simulink model "ESPp_linear_stiff"  (R2020b)
settings: Solver=ode8  StartTime=0.0  StopTime=T  FixedStep=0.001  RelTol=1e-3
values from neighbouring files (symbols this model uses):
  D = diag([d_par d_par d_par])    [main.m]    (also in main_linear.m)
  F = 1000*[-sin(q0(1)+q0(2)+q0(3)); cos(q0(1)+q0(2)+q0(3))]    [main.m]    (also in main_linear.m)
  invB = inv(B)    [main.m]    (also in main_linear.m)
  Kd = diag([500 500 500])    [main.m]    (also in main_linear.m = diag([kd_par kd_par kd_par]))
  Kp = diag([800 800 800])    [main.m]    (also in main_linear.m = diag([kp_par kp_par kp_par]))
  link = 3    [main.m]    (also in main_linear.m)
  motor = [I_m*k_r^2, k]    [main.m]    (also in main_linear.m = [I_m*k_r^2, k, k_new])
  param = [m mm d I g0]'    [main.m]    (also in main_linear.m)
  q0 = qd    [main.m]    (also in main_linear.m)
  qd = [pi/2; 0; 0]    [main.m]    (also in main_linear.m = [pi/3; -pi/7; pi/4])
  qd0 = [0; 0; 0]    [main.m]    (also in main_linear.m)
  qd_2dot = [0; 0; 0]    [main.m]    (also in main_linear.m)
  qd_3dot = [0; 0; 0]    [main.m]    (also in main_linear.m)
  qd_4dot = [0; 0; 0]    [main.m]    (also in main_linear.m)
  qd_dot = [0; 0; 0]    [main.m]    (also in main_linear.m)
  T1 = 2    [main.m]    (also in main_linear.m)
  T2 = 3    [main.m]    (also in main_linear.m)
  theta0 = q0    [main.m]    (also in main_linear.m)
  thetad0 = [0; 0; 0]    [main.m]    (also in main_linear.m)
settings Model: Creator=lorenzo  LastModifiedBy=lorenzo

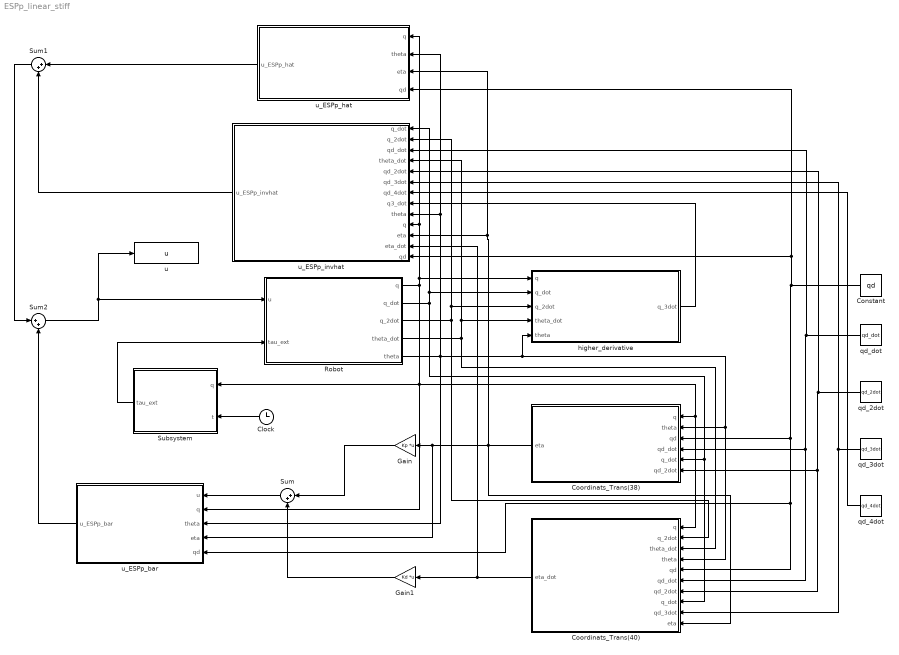
== system ESPp_linear_stiff ==
  Clock : Clock
  Constant : Constant  Value=qd  VectorParams1D=off
  Coordinats_Trans(38) : Subsystem
  Coordinats_Trans(40) : Subsystem
  Gain : Gain  Gain=Kp  Multiplication=Matrix(K*u) (u vector)
  Gain1 : Gain  Gain=Kd  Multiplication=Matrix(K*u) (u vector)
  Robot : Subsystem
  Subsystem : Subsystem
  Sum : Sum  Inputs=|++
  Sum1 : Sum  Inputs=|++
  Sum2 : Sum  Inputs=|++
  higher_derivative : Subsystem
  qd_2dot : Constant  Value=qd_2dot  VectorParams1D=off
  qd_3dot : Constant  Value=qd_3dot  VectorParams1D=off
  qd_4dot : Constant  Value=qd_4dot  VectorParams1D=off
  qd_dot : Constant  Value=qd_dot  VectorParams1D=off
  u : ToWorkspace  VariableName=u  SampleTime=-1
  u_ESPp_bar : Subsystem
  u_ESPp_hat : Subsystem
  u_ESPp_invhat : Subsystem
  wires:
  Robot/1(q) -> u_ESPp_hat/1("q "), u_ESPp_invhat/10("q "), higher_derivative/1("q "), Subsystem/1(q), Coordinats_Trans(40)/1(q), Coordinats_Trans(38)/1(q), u_ESPp_bar/2(q)
  Robot/2(q_dot) -> u_ESPp_invhat/1(q_dot), higher_derivative/2(q_dot), Coordinats_Trans(40)/8(q_dot), Coordinats_Trans(38)/5(" q_dot")
  Robot/3(q_2dot) -> higher_derivative/3(q_2dot), u_ESPp_invhat/2(q_2dot), Coordinats_Trans(40)/2(q_2dot)
  Robot/4("theta_dot ") -> u_ESPp_invhat/4(theta_dot), higher_derivative/4(theta_dot), Coordinats_Trans(40)/3(theta_dot)
  Coordinats_Trans(40)/1(eta_dot) -> u_ESPp_invhat/12(eta_dot), Gain1/1
  Coordinats_Trans(38)/1(eta) -> Coordinats_Trans(40)/10(eta), u_ESPp_hat/3(eta), u_ESPp_invhat/11(eta), u_ESPp_bar/4(eta), Gain/1
  Gain/1 -> Sum/1
  Gain1/1 -> Sum/2
  Sum2/1 -> u/1, Robot/1(u)
  u_ESPp_hat/1(u_ESPp_hat) -> Sum1/1
  u_ESPp_invhat/1(u_ESPp_invhat) -> Sum1/2
  Sum1/1 -> Sum2/1
  higher_derivative/1(q_3dot) -> u_ESPp_invhat/8(q3_dot)
  Robot/5(theta) -> u_ESPp_bar/3(theta), u_ESPp_invhat/9(theta), u_ESPp_hat/2(theta), higher_derivative/5(theta), Coordinats_Trans(38)/2(theta), Coordinats_Trans(40)/4(" theta")
  Sum/1 -> u_ESPp_bar/1(u)
  u_ESPp_bar/1(u_ESPp_bar) -> Sum2/2
  qd_2dot/1 -> u_ESPp_invhat/5(qd_2dot), Coordinats_Trans(40)/7(qd_2dot), Coordinats_Trans(38)/6(qd_2dot)
  qd_3dot/1 -> Coordinats_Trans(40)/9(qd_3dot), u_ESPp_invhat/6(qd_3dot)
  Constant/1 -> u_ESPp_invhat/13(qd), u_ESPp_hat/4(qd), u_ESPp_bar/5(qd), Coordinats_Trans(40)/5(qd), Coordinats_Trans(38)/3(" qd")
  qd_dot/1 -> u_ESPp_invhat/3(qd_dot), Coordinats_Trans(40)/6(qd_dot), Coordinats_Trans(38)/4(" qd_dot")
  qd_4dot/1 -> u_ESPp_invhat/7(qd_4dot)
  Subsystem/1(tau_ext) -> Robot/2(tau_ext)
  Clock/1 -> Subsystem/2(t)

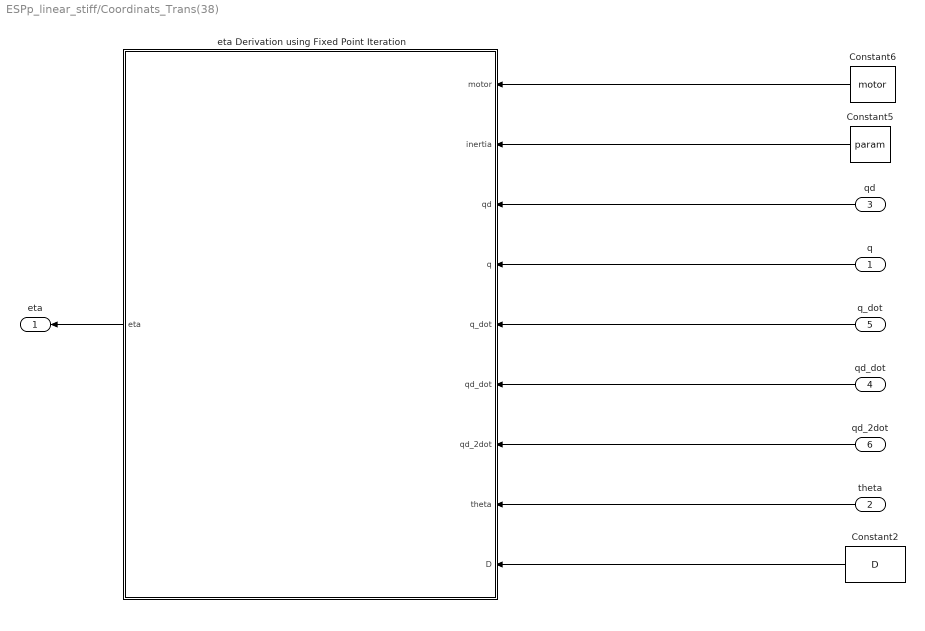
== system ESPp_linear_stiff/Coordinats_Trans(38) ==
  q : Inport
  theta : Inport  Port=2
  " qd" : Inport  Port=3
  " qd_dot" : Inport  Port=4
  " q_dot" : Inport  Port=5
  qd_2dot : Inport  Port=6
  Constant2 : Constant  Value=D  VectorParams1D=off
  Constant5 : Constant  Value=param  VectorParams1D=off
  Constant6 : Constant  Value=motor  VectorParams1D=off
  eta Derivation using Fixed Point Iteration : MATLAB Function  TreatAsAtomicUnit=on
  eta : Outport
  wires:
  Constant5/1 -> eta Derivation using Fixed Point Iteration/2(inertia)
  eta Derivation using Fixed Point Iteration/1(eta) -> eta/1
  theta/1 -> eta Derivation using Fixed Point Iteration/8(theta)
  Constant6/1 -> eta Derivation using Fixed Point Iteration/1(motor)
  q/1 -> eta Derivation using Fixed Point Iteration/4(q)
  " qd"/1 -> eta Derivation using Fixed Point Iteration/3(qd)
  " qd_dot"/1 -> eta Derivation using Fixed Point Iteration/6(qd_dot)
  " q_dot"/1 -> eta Derivation using Fixed Point Iteration/5(q_dot)
  qd_2dot/1 -> eta Derivation using Fixed Point Iteration/7(qd_2dot)
  Constant2/1 -> eta Derivation using Fixed Point Iteration/9(D)

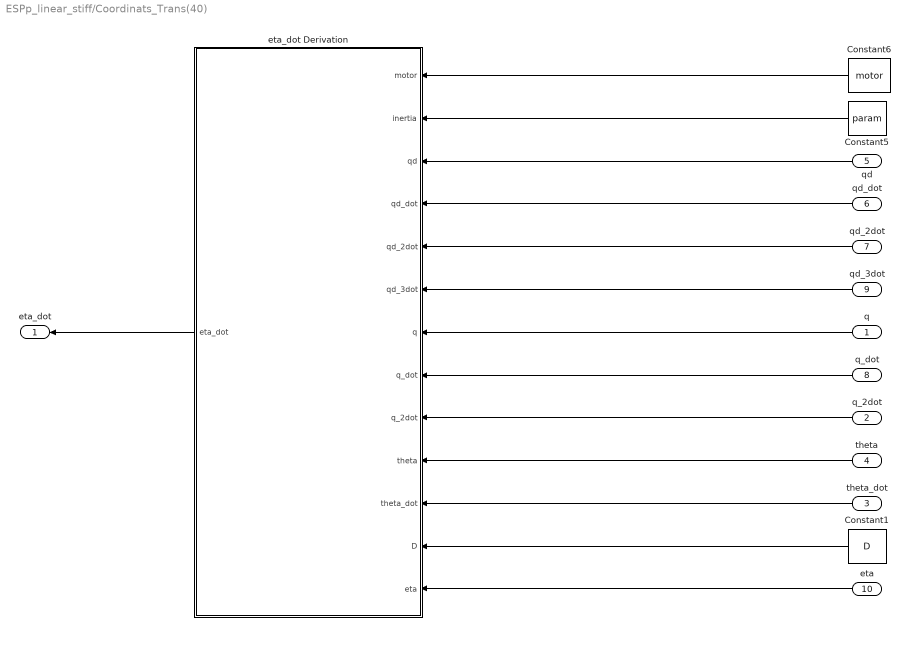
== system ESPp_linear_stiff/Coordinats_Trans(40) ==
  q : Inport
  q_2dot : Inport  Port=2
  theta_dot : Inport  Port=3
  " theta" : Inport  Port=4
  qd : Inport  Port=5
  qd_dot : Inport  Port=6
  qd_2dot : Inport  Port=7
  q_dot : Inport  Port=8
  qd_3dot : Inport  Port=9
  eta : Inport  Port=10
  Constant1 : Constant  Value=D  VectorParams1D=off
  Constant5 : Constant  Value=param  VectorParams1D=off
  Constant6 : Constant  Value=motor  VectorParams1D=off
  eta_dot Derivation : MATLAB Function  TreatAsAtomicUnit=on
  eta_dot : Outport
  wires:
  Constant5/1 -> eta_dot Derivation/2(inertia)
  eta_dot Derivation/1(eta_dot) -> eta_dot/1
  Constant6/1 -> eta_dot Derivation/1(motor)
  qd/1 -> eta_dot Derivation/3(qd)
  qd_dot/1 -> eta_dot Derivation/4(qd_dot)
  qd_2dot/1 -> eta_dot Derivation/5(qd_2dot)
  q/1 -> eta_dot Derivation/7(q)
  q_dot/1 -> eta_dot Derivation/8(q_dot)
  q_2dot/1 -> eta_dot Derivation/9(q_2dot)
  " theta"/1 -> eta_dot Derivation/10(theta)
  theta_dot/1 -> eta_dot Derivation/11(theta_dot)
  qd_3dot/1 -> eta_dot Derivation/6(qd_3dot)
  Constant1/1 -> eta_dot Derivation/12(D)
  eta/1 -> eta_dot Derivation/13(eta)

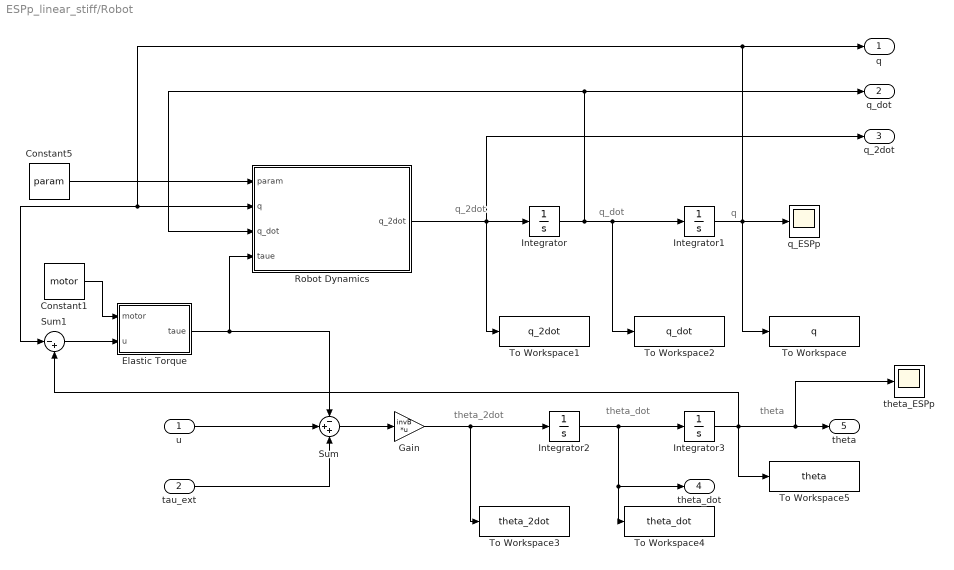
== system ESPp_linear_stiff/Robot ==
  note: theta_2dot
  note: q_dot
  note: theta_dot
  note: q
  note: q_2dot
  note: theta
  u : Inport
  tau_ext : Inport  Port=2
  Constant1 : Constant  Value=motor  VectorParams1D=off
  Constant5 : Constant  Value=param  VectorParams1D=off
  Elastic Torque : MATLAB Function  TreatAsAtomicUnit=on
  Gain : Gain  Gain=invB  Multiplication=Matrix(K*u)
  Integrator : Integrator  InitialCondition=qd0
  Integrator1 : Integrator  InitialCondition=q0
  Integrator2 : Integrator  InitialCondition=thetad0
  Integrator3 : Integrator  InitialCondition=theta0
  Robot Dynamics : MATLAB Function  TreatAsAtomicUnit=on
  Sum : Sum  Inputs=-++
  Sum1 : Sum  Inputs=|-+
  To Workspace : ToWorkspace  VariableName=q  SampleTime=-1
  To Workspace1 : ToWorkspace  VariableName=q_2dot  SampleTime=-1
  To Workspace2 : ToWorkspace  VariableName=q_dot  SampleTime=-1
  To Workspace3 : ToWorkspace  VariableName=theta_2dot  SampleTime=-1
  To Workspace4 : ToWorkspace  VariableName=theta_dot  SampleTime=-1
  To Workspace5 : ToWorkspace  VariableName=theta  SampleTime=-1
  q_ESPp : Scope
  theta_ESPp : Scope
  q : Outport
  q_dot : Outport  Port=2
  q_2dot : Outport  Port=3
  "theta_dot " : Outport  Port=4
  theta : Outport  Port=5
  wires:
  Sum1/1 -> Elastic Torque/2(u)
  Robot Dynamics/1(q_2dot) -> To Workspace1/1, q_2dot/1, Integrator/1
  Constant5/1 -> Robot Dynamics/1(param)
  Elastic Torque/1(taue) -> Sum/1, Robot Dynamics/4(taue)
  Sum/1 -> Gain/1
  Integrator1/1 -> Sum1/1, Robot Dynamics/2(q), q/1, q_ESPp/1, To Workspace/1
  Gain/1 -> To Workspace3/1, Integrator2/1
  Integrator/1 -> q_dot/1, Robot Dynamics/3(q_dot), To Workspace2/1, Integrator1/1
  u/1 -> Sum/2
  Constant1/1 -> Elastic Torque/1(motor)
  Integrator2/1 -> To Workspace4/1, "theta_dot "/1, Integrator3/1
  tau_ext/1 -> Sum/3
  Integrator3/1 -> To Workspace5/1, theta_ESPp/1, theta/1, Sum1/2

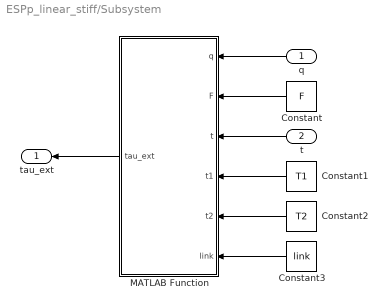
== system ESPp_linear_stiff/Subsystem ==
  q : Inport
  t : Inport  Port=2
  Constant : Constant  Value=F  VectorParams1D=off
  Constant1 : Constant  Value=T1  VectorParams1D=off
  Constant2 : Constant  Value=T2  VectorParams1D=off
  Constant3 : Constant  Value=link  VectorParams1D=off
  MATLAB Function : MATLAB Function  TreatAsAtomicUnit=on
  tau_ext : Outport
  wires:
  q/1 -> MATLAB Function/1(q)
  t/1 -> MATLAB Function/3(t)
  Constant1/1 -> MATLAB Function/4(t1)
  MATLAB Function/1(tau_ext) -> tau_ext/1
  Constant2/1 -> MATLAB Function/5(t2)
  Constant3/1 -> MATLAB Function/6(link)
  Constant/1 -> MATLAB Function/2(F)

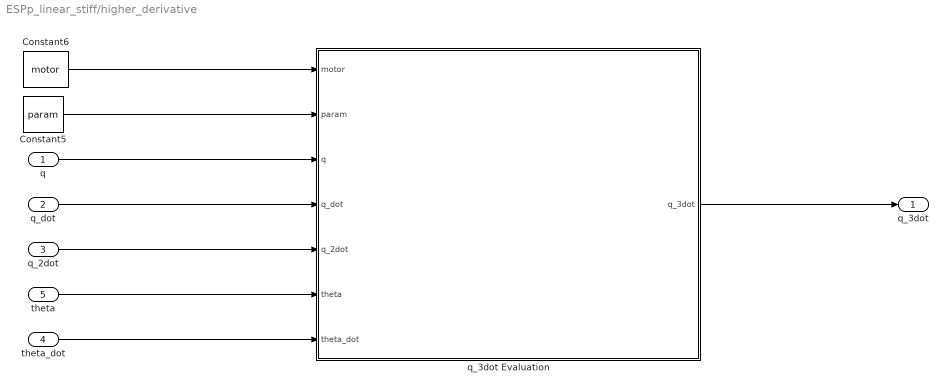
== system ESPp_linear_stiff/higher_derivative ==
  "q " : Inport
  q_dot : Inport  Port=2
  q_2dot : Inport  Port=3
  theta_dot : Inport  Port=4
  theta : Inport  Port=5
  Constant5 : Constant  Value=param  VectorParams1D=off
  Constant6 : Constant  Value=motor  VectorParams1D=off
  q_3dot Evaluation : MATLAB Function  TreatAsAtomicUnit=on
  q_3dot : Outport
  wires:
  Constant5/1 -> q_3dot Evaluation/2(param)
  q_dot/1 -> q_3dot Evaluation/4(q_dot)
  q_3dot Evaluation/1(q_3dot) -> q_3dot/1
  theta_dot/1 -> q_3dot Evaluation/7(theta_dot)
  q_2dot/1 -> q_3dot Evaluation/5(q_2dot)
  "q "/1 -> q_3dot Evaluation/3(q)
  Constant6/1 -> q_3dot Evaluation/1(motor)
  theta/1 -> q_3dot Evaluation/6(theta)

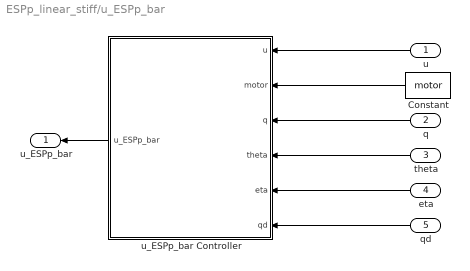
== system ESPp_linear_stiff/u_ESPp_bar ==
  u : Inport
  q : Inport  Port=2
  theta : Inport  Port=3
  eta : Inport  Port=4
  qd : Inport  Port=5
  Constant : Constant  Value=motor  VectorParams1D=off
  u_ESPp_bar Controller : MATLAB Function  TreatAsAtomicUnit=on
  u_ESPp_bar : Outport
  wires:
  eta/1 -> u_ESPp_bar Controller/5(eta)
  Constant/1 -> u_ESPp_bar Controller/2(motor)
  u_ESPp_bar Controller/1(u_ESPp_bar) -> u_ESPp_bar/1
  u/1 -> u_ESPp_bar Controller/1(u)
  theta/1 -> u_ESPp_bar Controller/4(theta)
  q/1 -> u_ESPp_bar Controller/3(q)
  qd/1 -> u_ESPp_bar Controller/6(qd)

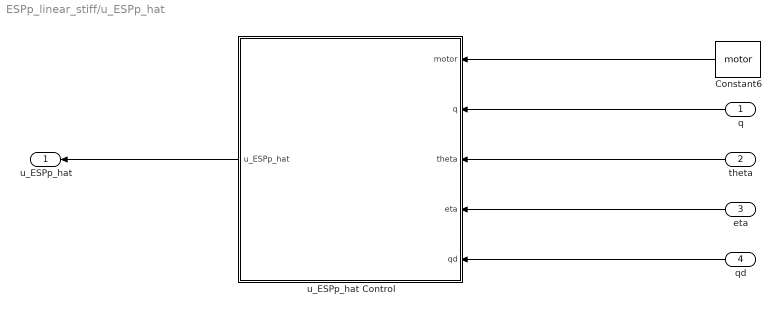
== system ESPp_linear_stiff/u_ESPp_hat ==
  "q " : Inport
  theta : Inport  Port=2
  eta : Inport  Port=3
  qd : Inport  Port=4
  Constant6 : Constant  Value=motor  VectorParams1D=off
  u_ESPp_hat Control : MATLAB Function  TreatAsAtomicUnit=on
  u_ESPp_hat : Outport
  wires:
  u_ESPp_hat Control/1(u_ESPp_hat) -> u_ESPp_hat/1
  theta/1 -> u_ESPp_hat Control/3(theta)
  "q "/1 -> u_ESPp_hat Control/2(q)
  Constant6/1 -> u_ESPp_hat Control/1(motor)
  eta/1 -> u_ESPp_hat Control/4(eta)
  qd/1 -> u_ESPp_hat Control/5(qd)

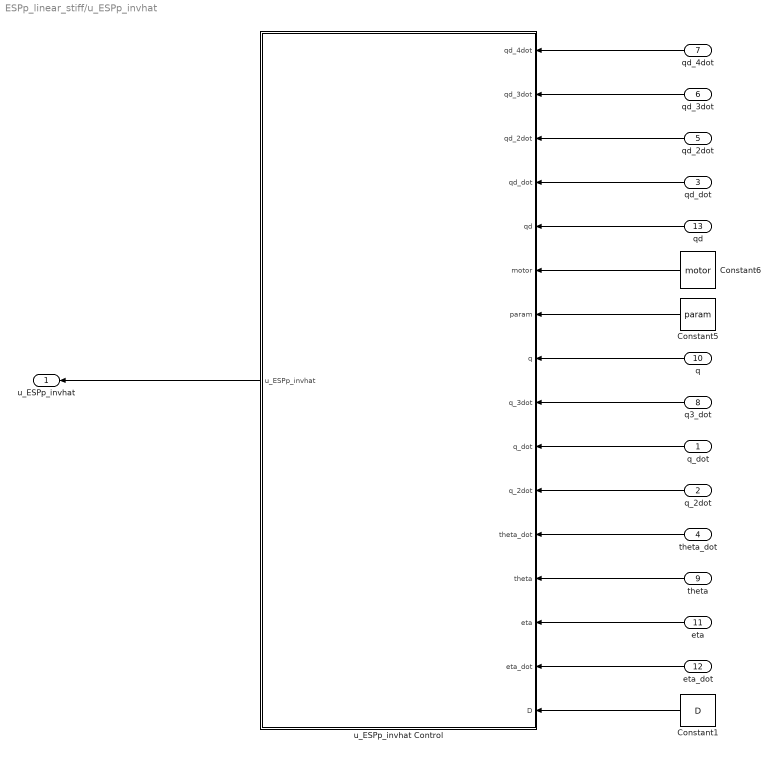
== system ESPp_linear_stiff/u_ESPp_invhat ==
  q_dot : Inport
  q_2dot : Inport  Port=2
  qd_dot : Inport  Port=3
  theta_dot : Inport  Port=4
  qd_2dot : Inport  Port=5
  qd_3dot : Inport  Port=6
  qd_4dot : Inport  Port=7
  q3_dot : Inport  Port=8
  theta : Inport  Port=9
  "q " : Inport  Port=10
  eta : Inport  Port=11
  eta_dot : Inport  Port=12
  qd : Inport  Port=13
  Constant1 : Constant  Value=D  VectorParams1D=off
  Constant5 : Constant  Value=param  VectorParams1D=off
  Constant6 : Constant  Value=motor  VectorParams1D=off
  u_ESPp_invhat Control : MATLAB Function  TreatAsAtomicUnit=on
  u_ESPp_invhat : Outport
  wires:
  q_dot/1 -> u_ESPp_invhat Control/10(q_dot)
  u_ESPp_invhat Control/1(u_ESPp_invhat) -> u_ESPp_invhat/1
  theta_dot/1 -> u_ESPp_invhat Control/12(theta_dot)
  q_2dot/1 -> u_ESPp_invhat Control/11(q_2dot)
  theta/1 -> u_ESPp_invhat Control/13(theta)
  "q "/1 -> u_ESPp_invhat Control/8(q)
  qd_2dot/1 -> u_ESPp_invhat Control/3(qd_2dot)
  qd_4dot/1 -> u_ESPp_invhat Control/1(qd_4dot)
  q3_dot/1 -> u_ESPp_invhat Control/9(q_3dot)
  Constant6/1 -> u_ESPp_invhat Control/6(motor)
  Constant5/1 -> u_ESPp_invhat Control/7(param)
  qd_3dot/1 -> u_ESPp_invhat Control/2(qd_3dot)
  qd_dot/1 -> u_ESPp_invhat Control/4(qd_dot)
  eta/1 -> u_ESPp_invhat Control/14(eta)
  eta_dot/1 -> u_ESPp_invhat Control/15(eta_dot)
  Constant1/1 -> u_ESPp_invhat Control/16(D)
  qd/1 -> u_ESPp_invhat Control/5(qd)

== matlab function ESPp_linear_stiff/u_ESPp_hat/u_ESPp_hat Control ==
  data: motor input; q input; u_ESPp_hat output; theta input; eta input; qd input
function u_ESPp_hat = u_ESPp_hat(motor, q, theta, eta, qd)
%% Iitialization of variables

% link side variables
q1 = q(1);
q2 = q(2);
q3 = q(3);

% motor side variables
theta1 = theta(1);
theta2 = theta(2);
theta3 = theta(3);

% new motor side variables
eta1 = eta(1);
eta2 = eta(2);
eta3 = eta(3);

% error variable
q_tilda = q - qd;

k = motor(2);     % stiffness
k_new = motor(3); % desired stiffness

% Stiffness vectors
% Psi1 = [k*sin(theta1-q1);k*sin(theta2-q2);k*sin(theta3-q3)];
% Psi2 = [k*sin(eta1-q_tilda(1));k*sin(eta2-q_tilda(2));k*sin(eta3-q_tilda(3))];
%Psi1 = k*[(theta1-q1)+(theta1-q1)^3; (theta2-q2)+(theta2-q2)^3; (theta3-q3)+(theta3-q3)^3];
%Psi2 = k*[(eta1-q_tilda(1))+(eta1-q_tilda(1))^3; (eta2-q_tilda(2))+(eta2-q_tilda(2))^3; (eta3-q_tilda(3))+(eta3-q_tilda(3))^3];

% Hermitian matrices
%K1 = diag(k*[1 + 3*(theta1-q1)^2; 1 + 3*(theta2-q2)^2; 1 + 3*(theta3-q3)^2]);
%K2 = diag(k*[1 + 3*(eta1-q_tilda(1))^2; 1 + 3*(eta2-q_tilda(2))^2; 1 + 3*(eta3-q_tilda(3))^2]);
K1 = diag([k; k; k]);
K2 = diag([k_new; k_new; k_new]);

invK1 = K1^-1;

%% Derivation of the control u_ESP_hat
A = invK1*K2;

% control
u_ESPp_hat = K1*(theta-q)-A'*K2*(eta-q_tilda);

== matlab function ESPp_linear_stiff/Robot/Elastic Torque ==
  data: motor input; u input; taue output
function taue = taue(motor, u)

k = motor(2);

% elastic torque
taue = k*[u(1); u(2); u(3)];

== matlab function ESPp_linear_stiff/Subsystem/MATLAB Function ==
  data: q input; tau_ext output; F input; t input; t1 input; t2 input; link input
function tau_ext = tau_ext(q, F, t, t1, t2, link)

tau_ext = zeros(3,1);

s1 = sin(q(1));
s12 = sin(q(1)+q(2));
s123 = sin(q(1)+q(2)+q(3));
c1 = cos(q(1));
c12 = cos(q(1)+q(2));
c123 = cos(q(1)+q(2)+q(3));
J = zeros(2, 3);

% choose the particular jacobian coordingly to where the external force
% acts
switch link
    case 1
        J = 0.5*[-s1 0 0; c1 0 0];
    case 2
        J = 0.5*[-s1-s12 -s12 0; c1+c12 c12 0];
    case 3
        J = 0.5*[-s1-s12-s123 -s12-s123 -s123; c1+c12+c123 c12+c123 c123];
end

if t>=t1 && t<=t2
    tau_ext = -J'*F;
end

== matlab function ESPp_linear_stiff/higher_derivative/q_3dot Evaluation ==
  data: motor input; param input; q input; q_3dot output size=[3 1]; q_dot input; q_2dot input; theta input; theta_dot input
function q_3dot = q_3dot(motor, param, q, q_dot, q_2dot, theta, theta_dot)
%% Initialization of the variables

% link variables
q1 = q(1);
q2 = q(2);
q3 = q(3);

q1d = q_dot(1);
q2d = q_dot(2);
q3d = q_dot(3);

q1dd = q_2dot(1);
q2dd = q_2dot(2);
q3dd = q_2dot(3);

% motor variables
theta1 = theta(1);
theta2 = theta(2);
theta3 = theta(3);

k = motor(2);       % stiffness
k_new = motor(3); %desired stiffness

%% Dynamical Parameters

% masses of the links
m1 = param(1);
m2 = m1;
m3 = m1;

% masses of the motors
m1m = param(2);
m2m = m1m;
m3m = m1m;

% distance from the CoM
d1 = param(3);
d2 = d1;
d3 = d1;

% inertia of the links
I1 = param(4);
I2 = I1;
I3 = I1;

% gravity acceleration
g0 = param(5);

a1 = m3*d3^2+I3;
a2 = m3*d3;
a3 = d3*m3;
a4 = I2+I3+d2^2*m2+d3^2*m3+m3+m3m;
a5 = m2*d2+m3m+m3;
a6 = I1+I2+I3+d1^2*m1+d2^2*m2+d3^2*m3+m1+m3+m3+m2m+m3m+m3m;

%% Inertia Matrix and its Derivatives

m11 = a6+2*a3*cos(q2+q3)+2*a5*cos(q2)+2*a2*cos(q3);
m12 = a4+a3*cos(q2+q3)+2*a2*cos(q3)+a5*cos(q2);
m13 = a1+a2*cos(q3)+a3*cos(q2+q3);
m21 = m12;
m22 = a4+2*a2*cos(q3);
m23 = a1+a2*cos(q3);
m31 = m13;
m32 = m23;
m33 = a1;

M = [m11 m12 m13;
    m21 m22 m23;
    m31 m32 m33];

M_dot = [ - 2*a3*sin(q2 + q3)*(q2d + q3d) - 2*a2*q3d*sin(q3) - 2*a5*q2d*sin(q2), - a3*sin(q2 + q3)*(q2d + q3d) - 2*a2*q3d*sin(q3) - a5*q2d*sin(q2), - a3*sin(q2 + q3)*(q2d + q3d) - a2*q3d*sin(q3);
     - a3*sin(q2 + q3)*(q2d + q3d) - 2*a2*q3d*sin(q3) - a5*q2d*sin(q2),                                                 -2*a2*q3d*sin(q3),                                -a2*q3d*sin(q3);
                        - a3*sin(q2 + q3)*(q2d + q3d) - a2*q3d*sin(q3),                                                   -a2*q3d*sin(q3),                                              0];
                    
%% gravity term

l1 = 1;
l2 = 1;

g = [g0*m2*(d2*cos(q1 + q2) + l1*cos(q1)) + g0*m3*(l2*cos(q1 + q2) + d3*cos(q1 + q2 + q3) + l1*cos(q1)) + d1*g0*m1*cos(q1);
                                                g0*m3*(l2*cos(q1 + q2) + d3*cos(q1 + q2 + q3)) + d2*g0*m2*cos(q1 + q2);
                                                                                            d3*g0*m3*cos(q1 + q2 + q3)];


g_dot = [ - g0*m2*(l1*q1d*sin(q1) + d2*sin(q1 + q2)*(q1d + q2d)) - g0*m3*(l1*q1d*sin(q1) + d3*sin(q1 + q2 + q3)*(q1d + q2d + q3d) + l2*sin(q1 + q2)*(q1d + q2d)) - d1*g0*m1*q1d*sin(q1);
                                                            - g0*m3*(d3*sin(q1 + q2 + q3)*(q1d + q2d + q3d) + l2*sin(q1 + q2)*(q1d + q2d)) - d2*g0*m2*sin(q1 + q2)*(q1d + q2d);
                                                                                                                                 -d3*g0*m3*sin(q1 + q2 + q3)*(q1d + q2d + q3d)];

%% Coriolis Terms and its Derivatives

S11 = - q3d*(a3*sin(q2 + q3) + a2*sin(q3)) - q2d*(a3*sin(q2 + q3) + a5*sin(q2));
S12 = - q1d*(a3*sin(q2 + q3) + a5*sin(q2)) - q3d*(a3*sin(q2 + q3) + a2*sin(q3)) - q2d*(a3*sin(q2 + q3) + a5*sin(q2));
S13 = - q1d*(a3*sin(q2 + q3) + a2*sin(q3)) - q2d*(a3*sin(q2 + q3) + a2*sin(q3)) - q3d*(a3*sin(q2 + q3) + a2*sin(q3));
S21 = q1d*(a3*sin(q2 + q3) + a5*sin(q2)) - a2*q3d*sin(q3);
S22 = -a2*q3d*sin(q3);
S23 = - a2*q1d*sin(q3) - a2*q2d*sin(q3) - a2*q3d*sin(q3);
S31 = q1d*(a3*sin(q2 + q3) + a2*sin(q3)) + a2*q2d*sin(q3);
S32 = a2*q1d*sin(q3) + a2*q2d*sin(q3);
S33 = 0;

C = [S11 S12 S13;
    S21 S22 S23;
    S31 S32 S33];

C_dot = [- q2d*(a3*cos(q2 + q3)*(q2d + q3d) + a5*q2d*cos(q2)) - q3d*(a3*cos(q2 + q3)*(q2d + q3d) + a2*q3d*cos(q3)) - q3dd*(a3*sin(q2 + q3) + a2*sin(q3)) - q2dd*(a3*sin(q2 + q3) + a5*sin(q2)), - q1d*(a3*cos(q2 + q3)*(q2d + q3d) + a5*q2d*cos(q2)) - q2d*(a3*cos(q2 + q3)*(q2d + q3d) + a5*q2d*cos(q2)) - q3d*(a3*cos(q2 + q3)*(q2d + q3d) + a2*q3d*cos(q3)) - q1dd*(a3*sin(q2 + q3) + a5*sin(q2)) - q3dd*(a3*sin(q2 + q3) + a2*sin(q3)) - q2dd*(a3*sin(q2 + q3) + a5*sin(q2)), - q1d*(a3*cos(q2 + q3)*(q2d + q3d) + a2*q3d*cos(q3)) - q2d*(a3*cos(q2 + q3)*(q2d + q3d) + a2*q3d*cos(q3)) - q3d*(a3*cos(q2 + q3)*(q2d + q3d) + a2*q3d*cos(q3)) - q1dd*(a3*sin(q2 + q3) + a2*sin(q3)) - q2dd*(a3*sin(q2 + q3) + a2*sin(q3)) - q3dd*(a3*sin(q2 + q3) + a2*sin(q3))
                                                        q1d*(a3*cos(q2 + q3)*(q2d + q3d) + a5*q2d*cos(q2)) + q1dd*(a3*sin(q2 + q3) + a5*sin(q2)) - a2*q3d^2*cos(q3) - a2*q3dd*sin(q3),                                                                                                                                                                                                                                               -a2*(cos(q3)*q3d^2 + q3dd*sin(q3)),                                                                                                                                                                             -a2*(q1dd*sin(q3) + q2dd*sin(q3) + q3dd*sin(q3) + q3d^2*cos(q3) + q1d*q3d*cos(q3) + q2d*q3d*cos(q3))
                                                      q1d*(a3*cos(q2 + q3)*(q2d + q3d) + a2*q3d*cos(q3)) + q1dd*(a3*sin(q2 + q3) + a2*sin(q3)) + a2*q2dd*sin(q3) + a2*q2d*q3d*cos(q3),                                                                                                                                                                                                             a2*(q1dd*sin(q3) + q2dd*sin(q3) + q1d*q3d*cos(q3) + q2d*q3d*cos(q3)),                                                                                                                                                                                                                                                                                0];

%% Compuation of q_3dot

% Stiffness vector
Psi1 = k*[(theta1-q1); (theta2-q2); (theta3-q3)];

% Hermitian matrices
%K1 = diag(k*[1 + 3*(theta1-q1)^2; 1 + 3*(theta2-q2)^2; 1 + 3*(theta3-q3)^2]);
K1 = diag([k,k,k]);

delta = Psi1-C*q_dot-g;

q_3dot = -inv(M)*M_dot*inv(M)*delta+inv(M)*(K1*(theta_dot-q_dot)-C_dot*q_dot-C*q_2dot-g_dot);

== matlab function ESPp_linear_stiff/Coordinats_Trans(38)/eta Derivation using Fixed Point Iteration ==
  data: motor input; inertia input; qd input; q input; q_dot input; qd_dot input; qd_2dot input; eta output size=[3 1]; theta input; D input
function eta = eta(motor, inertia, qd, q, q_dot, qd_dot, qd_2dot, theta, D)
%% Initialization of the variables

% link variables
q1 = q(1);
q2 = q(2);
q3 = q(3);

dq1 = q_dot(1);
dq2 = q_dot(2);
dq3 = q_dot(3);

% q_tilda and derivatives
q_tilda = q - qd;
q_dot_tilda = q_dot - qd_dot;

k = motor(2);   % stiffness
k_new = motor(3); % desired stiffness

% Stiffness matrix 
%Psi1 = [k*(theta(1)-q(1)-(theta(1)-q(1))^3);k*(theta(2)-q(2)-(theta(2)-q(2))^3);k*(theta(3)-q(3)-(theta(3)-q(3))^3)];
Psi1 = [k*(theta(1)-q(1)); k*(theta(2)-q(2)); k*(theta(3)-q(3))]; 

K1 = diag([k; k; k]);
K2 = diag([k_new; k_new; k_new]);
invK2 = K2^-1;

%% dynamic parameters

% masses of the links
m1 = inertia(1);
m2 = m1;
m3 = m1;

% masses of the motors
m1m = inertia(2);
m2m = m1m;
m3m = m1m;

% distance from the CoMs
d1 = inertia(3);
d2 = d1;
d3 = d1;

% inertia of the links
I1 = inertia(4);
I2 = I1;
I3 = I1;

% gravity acceleration
g0 = inertia(5);

a1 = m3*d3^2+I3;
a2 = m3*d3;
a3 = d3*m3;
a4 = I2+I3+d2^2*m2+d3^2*m3+m3+m3m;
a5 = m2*d2+m3m+m3;
a6 = I1+I2+I3+d1^2*m1+d2^2*m2+d3^2*m3+m1+m3+m3+m2m+m3m+m3m;

%% Gravity Term

l1 = 1;
l2 = 1;

g = [g0*m2*(d2*cos(q1 + q2) + l1*cos(q1)) + g0*m3*(l2*cos(q1 + q2) + d3*cos(q1 + q2 + q3) + l1*cos(q1)) + d1*g0*m1*cos(q1);
                                                g0*m3*(l2*cos(q1 + q2) + d3*cos(q1 + q2 + q3)) + d2*g0*m2*cos(q1 + q2);
                                                                                            d3*g0*m3*cos(q1 + q2 + q3)];

%% Inertia Matrix

m11 = a6+2*a3*cos(q2+q3)+2*a5*cos(q2)+2*a2*cos(q3);
m12 = a4+a3*cos(q2+q3)+2*a2*cos(q3)+a5*cos(q2);
m13 = a1+a2*cos(q3)+a3*cos(q2+q3);
m21 = m12;
m22 = a4+2*a2*cos(q3);
m23 = a1+a2*cos(q3);
m31 = m13;
m32 = m23;
m33 = a1;

M = [m11 m12 m13;
    m21 m22 m23;
    m31 m32 m33];

%% Coriolis Term

S11 = - dq3*(a3*sin(q2 + q3) + a2*sin(q3)) - dq2*(a3*sin(q2 + q3) + a5*sin(q2));
S12 = - dq1*(a3*sin(q2 + q3) + a5*sin(q2)) - dq3*(a3*sin(q2 + q3) + a2*sin(q3)) - dq2*(a3*sin(q2 + q3) + a5*sin(q2));
S13 = - dq1*(a3*sin(q2 + q3) + a2*sin(q3)) - dq2*(a3*sin(q2 + q3) + a2*sin(q3)) - dq3*(a3*sin(q2 + q3) + a2*sin(q3));
S21 = dq1*(a3*sin(q2 + q3) + a5*sin(q2)) - a2*dq3*sin(q3);
S22 = -a2*dq3*sin(q3);
S23 = - a2*dq1*sin(q3) - a2*dq2*sin(q3) - a2*dq3*sin(q3);
S31 = dq1*(a3*sin(q2 + q3) + a2*sin(q3)) + a2*dq2*sin(q3);
S32 = a2*dq1*sin(q3) + a2*dq2*sin(q3);
S33 = 0;

C = [S11 S12 S13;
    S21 S22 S23;
    S31 S32 S33];

%% Evaluate Eta using Fixed Point Iteration

% n = gravity + damping*q_dot + Inertia*q_2dot + Coriolis*q_dot
n = g - D*q_dot_tilda + M*qd_2dot + C*qd_dot;

eta = invK2*K1*(theta-q) - invK2*n + q_tilda;

% Psi2 = Psi1 - n;
% 
% % initialize the algorithm
% eta = zeros(3, 1);
% coder.extrinsic('comp_eta');
% 
% eta0 = fpi_params(1);
% eps = fpi_params(2);
% max_it = fpi_params(3);
% 
% eta = comp_eta(Psi2, eta0, k, q_tilda);

% for i = 1:3
%     
%     % initial guess
%     eta_temp = eta0;
%     
%     % initialization of variables for the while loop
%     j = 1;
%     fun = 2*eps;
%     
%     % stops if we reach the maximum number of iteration or if we have a
%     % sufficiently small error
%     while (j < max_it) && (fun > eps)
%         
%         % error between function evaluated in the guess and the real value
%         fun = -sin(eta_temp - q_tilda(i)) + 1/k*Psi2(i);
%         
%         % update theta value
%         eta_temp = eta_temp + fun;
%         
%         % true error
%         fun = abs(fun);
%         
%         j = j + 1;
%     end
%     
%     % assign the vaue of eta
%     eta(i) = eta_temp;
%     
% end

end

== matlab function ESPp_linear_stiff/Coordinats_Trans(40)/eta_dot Derivation ==
  data: motor input; inertia input; qd input; qd_dot input; qd_2dot input; qd_3dot input; q input; eta_dot output; q_dot input; q_2dot input; theta input; theta_dot input; D input; eta input
function eta_dot = eta_dot(motor, inertia, qd, qd_dot, qd_2dot, qd_3dot, q, q_dot, q_2dot, theta, theta_dot, D, eta)
%% Initialization of the variables

% link variables
q1 = q(1);
q2 = q(2);
q3 = q(3);

q1d = q_dot(1);
q2d = q_dot(2);
q3d = q_dot(3);

q1dd = q_2dot(1);
q2dd = q_2dot(2);
q3dd = q_2dot(3);

% q_tilda and derivatives
q_tilda = q - qd;
q_dot_tilda = q_dot - qd_dot;
q_2dot_tilda = q_2dot - qd_2dot;

% motor variables
theta1 = theta(1);
theta2 = theta(2);
theta3 = theta(3);

% new motor variables
eta1 = eta(1);
eta2 = eta(2);
eta3 = eta(3);

k = motor(2);   % stiffness
k_new = motor(3); % desired stiffness

%% Dynamic parameters

% masses of the links
m1 = inertia(1);
m2 = m1;
m3 = m1;

% masses of the motors
m1m = inertia(2);
m2m = m1m;
m3m = m1m;

% distance from the CoMs
d1 = inertia(3);
d2 = d1;
d3 = d1;

% inertia of the links
I1 = inertia(4);
I2 = I1;
I3 = I1;

% gravity acceleration
g0 = inertia(5);

a1 = m3*d3^2+I3;
a2 = m3*d3;
a3 = d3*m3;
a4 = I2+I3+d2^2*m2+d3^2*m3+m3+m3m;
a5 = m2*d2+m3m+m3;
a6 = I1+I2+I3+d1^2*m1+d2^2*m2+d3^2*m3+m1+m3+m3+m2m+m3m+m3m;

%% Inertia Matrix and its Derivatives

m11 = a6+2*a3*cos(q2+q3)+2*a5*cos(q2)+2*a2*cos(q3);
m12 = a4+a3*cos(q2+q3)+2*a2*cos(q3)+a5*cos(q2);
m13 = a1+a2*cos(q3)+a3*cos(q2+q3);
m21 = m12;
m22 = a4+2*a2*cos(q3);
m23 = a1+a2*cos(q3);
m31 = m13;
m32 = m23;
m33 = a1;

M = [m11 m12 m13;
    m21 m22 m23;
    m31 m32 m33];

M_dot = [- 2*a2*q3d*sin(q3) - 2*a5*q2d*sin(q2) - 2*a3*sin(q2 + q3)*(q2d + q3d), - 2*a2*q3d*sin(q3) - a5*q2d*sin(q2) - a3*sin(q2 + q3)*(q2d + q3d), - a2*q3d*sin(q3) - a3*sin(q2 + q3)*(q2d + q3d);
             - 2*a2*q3d*sin(q3) - a5*q2d*sin(q2) - a3*sin(q2 + q3)*(q2d + q3d),                                                          -2*a2*q3d*sin(q3),                                      -a2*q3d*sin(q3);
                                   - a2*q3d*sin(q3) - a3*sin(q2 + q3)*(q2d + q3d),                                                            -a2*q3d*sin(q3),                                                       0];

%% Gravity Term

l1 = 1;
l2 = 1;

g_dot = [ - g0*m2*(l1*q1d*sin(q1) + d2*sin(q1 + q2)*(q1d + q2d)) - g0*m3*(l1*q1d*sin(q1) + d3*sin(q1 + q2 + q3)*(q1d + q2d + q3d) + l2*sin(q1 + q2)*(q1d + q2d)) - d1*g0*m1*q1d*sin(q1);
                                                            - g0*m3*(d3*sin(q1 + q2 + q3)*(q1d + q2d + q3d) + l2*sin(q1 + q2)*(q1d + q2d)) - d2*g0*m2*sin(q1 + q2)*(q1d + q2d);
                                                                                                                                 -d3*g0*m3*sin(q1 + q2 + q3)*(q1d + q2d + q3d)];


%% Coriolis Terms and its Derivative

S11 = - q3d*(a3*sin(q2 + q3) + a2*sin(q3)) - q2d*(a3*sin(q2 + q3) + a5*sin(q2));
S12 = - q1d*(a3*sin(q2 + q3) + a5*sin(q2)) - q3d*(a3*sin(q2 + q3) + a2*sin(q3)) - q2d*(a3*sin(q2 + q3) + a5*sin(q2));
S13 = - q1d*(a3*sin(q2 + q3) + a2*sin(q3)) - q2d*(a3*sin(q2 + q3) + a2*sin(q3)) - q3d*(a3*sin(q2 + q3) + a2*sin(q3));
S21 = q1d*(a3*sin(q2 + q3) + a5*sin(q2)) - a2*q3d*sin(q3);
S22 = -a2*q3d*sin(q3);
S23 = - a2*q1d*sin(q3) - a2*q2d*sin(q3) - a2*q3d*sin(q3);
S31 = q1d*(a3*sin(q2 + q3) + a2*sin(q3)) + a2*q2d*sin(q3);
S32 = a2*q1d*sin(q3) + a2*q2d*sin(q3);
S33 = 0;

C = [S11 S12 S13;
    S21 S22 S23;
    S31 S32 S33];

C_dot = [- q2d*(a3*cos(q2 + q3)*(q2d + q3d) + a5*q2d*cos(q2)) - q3d*(a3*cos(q2 + q3)*(q2d + q3d) + a2*q3d*cos(q3)) - q3dd*(a3*sin(q2 + q3) + a2*sin(q3)) - q2dd*(a3*sin(q2 + q3) + a5*sin(q2)), - q1d*(a3*cos(q2 + q3)*(q2d + q3d) + a5*q2d*cos(q2)) - q2d*(a3*cos(q2 + q3)*(q2d + q3d) + a5*q2d*cos(q2)) - q3d*(a3*cos(q2 + q3)*(q2d + q3d) + a2*q3d*cos(q3)) - q1dd*(a3*sin(q2 + q3) + a5*sin(q2)) - q3dd*(a3*sin(q2 + q3) + a2*sin(q3)) - q2dd*(a3*sin(q2 + q3) + a5*sin(q2)), - q1d*(a3*cos(q2 + q3)*(q2d + q3d) + a2*q3d*cos(q3)) - q2d*(a3*cos(q2 + q3)*(q2d + q3d) + a2*q3d*cos(q3)) - q3d*(a3*cos(q2 + q3)*(q2d + q3d) + a2*q3d*cos(q3)) - q1dd*(a3*sin(q2 + q3) + a2*sin(q3)) - q2dd*(a3*sin(q2 + q3) + a2*sin(q3)) - q3dd*(a3*sin(q2 + q3) + a2*sin(q3))
                                                        q1d*(a3*cos(q2 + q3)*(q2d + q3d) + a5*q2d*cos(q2)) + q1dd*(a3*sin(q2 + q3) + a5*sin(q2)) - a2*q3d^2*cos(q3) - a2*q3dd*sin(q3),                                                                                                                                                                                                                                               -a2*(cos(q3)*q3d^2 + q3dd*sin(q3)),                                                                                                                                                                             -a2*(q1dd*sin(q3) + q2dd*sin(q3) + q3dd*sin(q3) + q3d^2*cos(q3) + q1d*q3d*cos(q3) + q2d*q3d*cos(q3))
                                                      q1d*(a3*cos(q2 + q3)*(q2d + q3d) + a2*q3d*cos(q3)) + q1dd*(a3*sin(q2 + q3) + a2*sin(q3)) + a2*q2dd*sin(q3) + a2*q2d*q3d*cos(q3),                                                                                                                                                                                                             a2*(q1dd*sin(q3) + q2dd*sin(q3) + q1d*q3d*cos(q3) + q2d*q3d*cos(q3)),                                                                                                                                                                                                                                                                                0];

%% Computation of eta_dot

% Hermitian matrices
%K1 = diag(k*[1 + 3*(theta1-q1)^2; 1 + 3*(theta2-q2)^2; 1 + 3*(theta3-q3)^2]);
%K2 = diag(k*[1 + 3*(eta1-q_tilda(1))^2; 1 + 3*(eta2-q_tilda(2))^2; 1 + 3*(eta3-q_tilda(3))^2]);

K1 = diag([k; k; k]);
K2 = diag([k_new; k_new; k_new]);

n_dot = g_dot - D*q_2dot_tilda + M_dot*qd_2dot + M*qd_3dot + C_dot*qd_dot + C*qd_2dot;

eta_dot = q_dot_tilda + K2^-1*(K1*(theta_dot - q_dot) - n_dot);

== matlab function ESPp_linear_stiff/u_ESPp_bar/u_ESPp_bar Controller ==
  data: u input; motor input; u_ESPp_bar output; q input; theta input; eta input; qd input
function u_ESPp_bar = u_ESPp_bar(u, motor, q, theta, eta, qd)
%% Initialization of the variables

% link variables
q1 = q(1);
q2 = q(2);
q3 = q(3);

% motor variables
theta1 = theta(1);
theta2 = theta(2);
theta3 = theta(3);

% new motor variables
eta1 = eta(1);
eta2 = eta(2);
eta3 = eta(3);

% error variables
q_tilda = q - qd;

k = motor(2);   % stiffness
k_new = motor(3); % desired stiffness

% Hermitian matrices
%K1 = diag(k*[1 + 3*(theta1-q1)^2; 1 + 3*(theta2-q2)^2; 1 + 3*(theta3-q3)^2]);
%K2 = diag(k*[1 + 3*(eta1-q_tilda(1))^2; 1 + 3*(eta2-q_tilda(2))^2; 1 + 3*(eta3-q_tilda(3))^2]);
K1 = diag([k; k; k]);
K2 = diag([k_new; k_new; k_new]);
invK1 = K1^-1;

%% Controller derivation

A = invK1*K2;

u_ESPp_bar = -(A')^-1*u;

== matlab function ESPp_linear_stiff/Robot/Robot Dynamics ==
  data: param input; q input; q_2dot output size=[3 1]; q_dot input; taue input
function q_2dot = q_2dot(param, q, q_dot, taue)
%% Initialization of the variables

% link variables
q1 = q(1);
q2 = q(2);
q3 = q(3);

q1d = q_dot(1);
q2d = q_dot(2);
q3d = q_dot(3);

% masses of the links
m1 = param(1);
m2 = m1;
m3 = m1;

% masses of the motors
m1m = param(2);
m2m = m1m;
m3m = m1m;

% distance from the CoMs
d1 = param(3);
d2 = d1;
d3 = d1;

% inertia of the links
I1 = param(4);
I2 = I1;
I3 = I1;

% acceleration of gravity
g0 = param(5);

a1 = m3*d3^2+I3;
a2 = m3*d3;
a3 = d3*m3;
a4 = I2+I3+d2^2*m2+d3^2*m3+m3+m3m;
a5 = m2*d2+m3m+m3;
a6 = I1+I2+I3+d1^2*m1+d2^2*m2+d3^2*m3+m1+m3+m3+m2m+m3m+m3m;

%% Inertia matrix

m11 = a6+2*a3*cos(q2+q3)+2*a5*cos(q2)+2*a2*cos(q3);
m12 = a4+a3*cos(q2+q3)+2*a2*cos(q3)+a5*cos(q2);
m13 = a1+a2*cos(q3)+a3*cos(q2+q3);
m21 = m12;
m22 = a4+2*a2*cos(q3);
m23 = a1+a2*cos(q3);
m31 = m13;
m32 = m23;
m33 = a1;

M = [m11 m12 m13;
    m21 m22 m23;
    m31 m32 m33];

%% Coriolis term

C = [- a3*q2d^2*sin(q2 + q3) - a3*q3d^2*sin(q2 + q3) - a2*q3d^2*sin(q3) - a5*q2d^2*sin(q2) - 2*a3*q1d*q2d*sin(q2 + q3) - 2*a3*q1d*q3d*sin(q2 + q3) - 2*a3*q2d*q3d*sin(q2 + q3) - 2*a2*q1d*q3d*sin(q3) - 2*a2*q2d*q3d*sin(q3) - 2*a5*q1d*q2d*sin(q2);
                                                                                                                                      a3*q1d^2*sin(q2 + q3) - a2*q3d^2*sin(q3) + a5*q1d^2*sin(q2) - 2*a2*q1d*q3d*sin(q3) - 2*a2*q2d*q3d*sin(q3);
                                                                                                                                                             a3*q1d^2*sin(q2 + q3) + a2*q1d^2*sin(q3) + a2*q2d^2*sin(q3) + 2*a2*q1d*q2d*sin(q3)];

%% Gravity term

l1 = 1;
l2 = 1;

g = [g0*m2*(d2*cos(q1 + q2) + l1*cos(q1)) + g0*m3*(l2*cos(q1 + q2) + d3*cos(q1 + q2 + q3) + l1*cos(q1)) + d1*g0*m1*cos(q1);
                                                g0*m3*(l2*cos(q1 + q2) + d3*cos(q1 + q2 + q3)) + d2*g0*m2*cos(q1 + q2);
                                                                                            d3*g0*m3*cos(q1 + q2 + q3)];

%% Evaluation of q_2dot

q_2dot = M^-1*(taue - C - g);

== matlab function ESPp_linear_stiff/u_ESPp_invhat/u_ESPp_invhat Control ==
  data: qd_4dot input; qd_3dot input; qd_2dot input; qd_dot input; qd input; motor input; param input; q input; q_3dot input; u_ESPp_invhat output; q_dot input; q_2dot input; theta_dot input; theta input; eta input; eta_dot input; D input
function u_ESPp_invhat = u_ESPp_invhat(qd_4dot, qd_3dot, qd_2dot, qd_dot, qd, motor, param, q, q_3dot, q_dot, q_2dot, theta_dot, theta, eta, eta_dot, D)
%% initialization of variables

% link variables
q1 = q(1);
q2 = q(2);
q3 = q(3);

q1d = q_dot(1);
q2d = q_dot(2);
q3d = q_dot(3);

q1dd = q_2dot(1);
q2dd = q_2dot(2);
q3dd = q_2dot(3);

q1ddd = q_3dot(1);
q2ddd = q_3dot(2);
q3ddd = q_3dot(3);

% motor variables
theta1 = theta(1);
theta2 = theta(2);
theta3 = theta(3);

dottheta1 = theta_dot(1);
dottheta2 = theta_dot(2);
dottheta3 = theta_dot(3);

% new motor variables
eta1 = eta(1);
eta2 = eta(2);
eta3 = eta(3);

doteta1 = eta_dot(1);
doteta2 = eta_dot(2);
doteta3 = eta_dot(3);

% q_tilda and derivatives
q_tilda = q - qd;
dot_q_tilda = q_dot - qd_dot;
ddot_q_tilda = q_2dot - qd_2dot;
dddot_q_tilda = q_3dot - qd_3dot;

%% Dynamic Parameters

b = motor(1);    % motor inertia
k = motor(2);    % stiffness
k_new = motor(3); % desired stiffness

% link masses
m1 = param(1);  
m2 = m1;
m3 = m1;

% motor masses
m1m = param(2);
m2m = m1m;
m3m = m1m;

% distance from the CoMs
d1 = param(3);
d2 = d1;
d3 = d1;

% inertia of the links
I1 = param(4);
I2 = I1;
I3 = I1;

% gravity acceleration
g0 = param(5);

a1 = m3*d3^2+I3;
a2 = m3*d3;
a3 = d3*m3;
a4 = I2+I3+d2^2*m2+d3^2*m3+m3+m3m;
a5 = m2*d2+m3m+m3;
a6 = I1+I2+I3+d1^2*m1+d2^2*m2+d3^2*m3+m1+m3+m3+m2m+m3m+m3m;

% Linear Inertia matrix motor
B = diag([b, b, b]);

% Hermitian matrices
K1 = diag([k; k; k]);
K2 = diag([k_new; k_new; k_new]);

%K1 = diag(k*[1 + 3*(theta1-q1)^2; 1 + 3*(theta2-q2)^2; 1 + 3*(theta3-q3)^2]);
%K2 = diag(k*[1 + 3*(eta1-q_tilda(1))^2; 1 + 3*(eta2-q_tilda(2))^2; 1 + 3*(eta3-q_tilda(3))^2]);
invK1 = K1^-1;

% % derivatives of Hermitian matrices
% dotK1 = diag(k*[(1 + 3*(theta1-q1)^2)*(dottheta1-q1d); (1 + 3*(theta2-q2)^2)*(dottheta2-q2d); (1 + 3*(theta3-q3)^2)*(dottheta3-q3d)]);
% dotK2 = diag(k*[(1 + 3*(eta1-q_tilda(1))^2)*(doteta1-dot_q_tilda(1)); (1 + 3*(eta2-q_tilda(2))^2)*(doteta2-dot_q_tilda(2)); (1 + 3*(eta3-q_tilda(3))^2)*(doteta3-dot_q_tilda(3))]);
% 
% dotinvK1 = -invK1*dotK1*invK1;

%% Inertia matrix and its Derivatives

m11 = a6+2*a3*cos(q2+q3)+2*a5*cos(q2)+2*a2*cos(q3);
m12 = a4+a3*cos(q2+q3)+2*a2*cos(q3)+a5*cos(q2);
m13 = a1+a2*cos(q3)+a3*cos(q2+q3);
m21 = m12;
m22 = a4+2*a2*cos(q3);
m23 = a1+a2*cos(q3);
m31 = m13;
m32 = m23;
m33 = a1;

M = [m11 m12 m13;
    m21 m22 m23;
    m31 m32 m33];

dotM = [ - 2*a3*sin(q2 + q3)*(q2d + q3d) - 2*a2*q3d*sin(q3) - 2*a5*q2d*sin(q2), - a3*sin(q2 + q3)*(q2d + q3d) - 2*a2*q3d*sin(q3) - a5*q2d*sin(q2), - a3*sin(q2 + q3)*(q2d + q3d) - a2*q3d*sin(q3);
     - a3*sin(q2 + q3)*(q2d + q3d) - 2*a2*q3d*sin(q3) - a5*q2d*sin(q2),                                                 -2*a2*q3d*sin(q3),                                -a2*q3d*sin(q3);
                        - a3*sin(q2 + q3)*(q2d + q3d) - a2*q3d*sin(q3),                                                   -a2*q3d*sin(q3),                                              0];
                    
ddotM = [ - 2*a2*q3d^2*cos(q3) - 2*a5*q2d^2*cos(q2) - 2*a3*sin(q2 + q3)*(q2dd + q3dd) - 2*a3*cos(q2 + q3)*(q2d + q3d)^2 - 2*a2*q3dd*sin(q3) - 2*a5*q2dd*sin(q2), - 2*a2*q3d^2*cos(q3) - a5*q2d^2*cos(q2) - a3*sin(q2 + q3)*(q2dd + q3dd) - a3*cos(q2 + q3)*(q2d + q3d)^2 - 2*a2*q3dd*sin(q3) - a5*q2dd*sin(q2), - a2*q3d^2*cos(q3) - a3*sin(q2 + q3)*(q2dd + q3dd) - a3*cos(q2 + q3)*(q2d + q3d)^2 - a2*q3dd*sin(q3);
         - 2*a2*q3d^2*cos(q3) - a5*q2d^2*cos(q2) - a3*sin(q2 + q3)*(q2dd + q3dd) - a3*cos(q2 + q3)*(q2d + q3d)^2 - 2*a2*q3dd*sin(q3) - a5*q2dd*sin(q2),                                                                                                      - 2*a2*cos(q3)*q3d^2 - 2*a2*q3dd*sin(q3),                                                                 - a2*cos(q3)*q3d^2 - a2*q3dd*sin(q3);
                                                  - a2*q3d^2*cos(q3) - a3*sin(q2 + q3)*(q2dd + q3dd) - a3*cos(q2 + q3)*(q2d + q3d)^2 - a2*q3dd*sin(q3),                                                                                                          - a2*cos(q3)*q3d^2 - a2*q3dd*sin(q3),                                                                                                    0];

%% Coriolis term and its Derivatives

S11 = - q3d*(a3*sin(q2 + q3) + a2*sin(q3)) - q2d*(a3*sin(q2 + q3) + a5*sin(q2));
S12 = - q1d*(a3*sin(q2 + q3) + a5*sin(q2)) - q3d*(a3*sin(q2 + q3) + a2*sin(q3)) - q2d*(a3*sin(q2 + q3) + a5*sin(q2));
S13 = - q1d*(a3*sin(q2 + q3) + a2*sin(q3)) - q2d*(a3*sin(q2 + q3) + a2*sin(q3)) - q3d*(a3*sin(q2 + q3) + a2*sin(q3));
S21 = q1d*(a3*sin(q2 + q3) + a5*sin(q2)) - a2*q3d*sin(q3);
S22 = -a2*q3d*sin(q3);
S23 = - a2*q1d*sin(q3) - a2*q2d*sin(q3) - a2*q3d*sin(q3);
S31 = q1d*(a3*sin(q2 + q3) + a2*sin(q3)) + a2*q2d*sin(q3);
S32 = a2*q1d*sin(q3) + a2*q2d*sin(q3);
S33 = 0;   

C = [S11 S12 S13;
    S21 S22 S23;
    S31 S32 S33];

dotC = [ - q2d*(a3*cos(q2 + q3)*(q2d + q3d) + a5*q2d*cos(q2)) - q3d*(a3*cos(q2 + q3)*(q2d + q3d) + a2*q3d*cos(q3)) - q3dd*(a3*sin(q2 + q3) + a2*sin(q3)) - q2dd*(a3*sin(q2 + q3) + a5*sin(q2)), - q1d*(a3*cos(q2 + q3)*(q2d + q3d) + a5*q2d*cos(q2)) - q2d*(a3*cos(q2 + q3)*(q2d + q3d) + a5*q2d*cos(q2)) - q3d*(a3*cos(q2 + q3)*(q2d + q3d) + a2*q3d*cos(q3)) - q1dd*(a3*sin(q2 + q3) + a5*sin(q2)) - q3dd*(a3*sin(q2 + q3) + a2*sin(q3)) - q2dd*(a3*sin(q2 + q3) + a5*sin(q2)), - q1d*(a3*cos(q2 + q3)*(q2d + q3d) + a2*q3d*cos(q3)) - q2d*(a3*cos(q2 + q3)*(q2d + q3d) + a2*q3d*cos(q3)) - q3d*(a3*cos(q2 + q3)*(q2d + q3d) + a2*q3d*cos(q3)) - q1dd*(a3*sin(q2 + q3) + a2*sin(q3)) - q2dd*(a3*sin(q2 + q3) + a2*sin(q3)) - q3dd*(a3*sin(q2 + q3) + a2*sin(q3));
                                                         q1d*(a3*cos(q2 + q3)*(q2d + q3d) + a5*q2d*cos(q2)) + q1dd*(a3*sin(q2 + q3) + a5*sin(q2)) - a2*q3d^2*cos(q3) - a2*q3dd*sin(q3),                                                                                                                                                                                                                                               -a2*(cos(q3)*q3d^2 + q3dd*sin(q3)),                                                                                                                                                                             -a2*(q1dd*sin(q3) + q2dd*sin(q3) + q3dd*sin(q3) + q3d^2*cos(q3) + q1d*q3d*cos(q3) + q2d*q3d*cos(q3));
                                                       q1d*(a3*cos(q2 + q3)*(q2d + q3d) + a2*q3d*cos(q3)) + q1dd*(a3*sin(q2 + q3) + a2*sin(q3)) + a2*q2dd*sin(q3) + a2*q2d*q3d*cos(q3),                                                                                                                                                                                                             a2*(q1dd*sin(q3) + q2dd*sin(q3) + q1d*q3d*cos(q3) + q2d*q3d*cos(q3)),                                                                                                                                                                                                                                                                                0];

ddotC = [ q3d*(a2*q3d^2*sin(q3) - a3*cos(q2 + q3)*(q2dd + q3dd) + a3*sin(q2 + q3)*(q2d + q3d)^2 - a2*q3dd*cos(q3)) - 2*q3dd*(a3*cos(q2 + q3)*(q2d + q3d) + a2*q3d*cos(q3)) - 2*q2dd*(a3*cos(q2 + q3)*(q2d + q3d) + a5*q2d*cos(q2)) + q2d*(a5*q2d^2*sin(q2) - a3*cos(q2 + q3)*(q2dd + q3dd) + a3*sin(q2 + q3)*(q2d + q3d)^2 - a5*q2dd*cos(q2)) - q3ddd*(a3*sin(q2 + q3) + a2*sin(q3)) - q2ddd*(a3*sin(q2 + q3) + a5*sin(q2)), q1d*(a5*q2d^2*sin(q2) - a3*cos(q2 + q3)*(q2dd + q3dd) + a3*sin(q2 + q3)*(q2d + q3d)^2 - a5*q2dd*cos(q2)) - 2*q2dd*(a3*cos(q2 + q3)*(q2d + q3d) + a5*q2d*cos(q2)) - 2*q3dd*(a3*cos(q2 + q3)*(q2d + q3d) + a2*q3d*cos(q3)) - 2*q1dd*(a3*cos(q2 + q3)*(q2d + q3d) + a5*q2d*cos(q2)) + q3d*(a2*q3d^2*sin(q3) - a3*cos(q2 + q3)*(q2dd + q3dd) + a3*sin(q2 + q3)*(q2d + q3d)^2 - a2*q3dd*cos(q3)) + q2d*(a5*q2d^2*sin(q2) - a3*cos(q2 + q3)*(q2dd + q3dd) + a3*sin(q2 + q3)*(q2d + q3d)^2 - a5*q2dd*cos(q2)) - q1ddd*(a3*sin(q2 + q3) + a5*sin(q2)) - q3ddd*(a3*sin(q2 + q3) + a2*sin(q3)) - q2ddd*(a3*sin(q2 + q3) + a5*sin(q2)), q1d*(a2*q3d^2*sin(q3) - a3*cos(q2 + q3)*(q2dd + q3dd) + a3*sin(q2 + q3)*(q2d + q3d)^2 - a2*q3dd*cos(q3)) - 2*q2dd*(a3*cos(q2 + q3)*(q2d + q3d) + a2*q3d*cos(q3)) - 2*q3dd*(a3*cos(q2 + q3)*(q2d + q3d) + a2*q3d*cos(q3)) - 2*q1dd*(a3*cos(q2 + q3)*(q2d + q3d) + a2*q3d*cos(q3)) + q2d*(a2*q3d^2*sin(q3) - a3*cos(q2 + q3)*(q2dd + q3dd) + a3*sin(q2 + q3)*(q2d + q3d)^2 - a2*q3dd*cos(q3)) + q3d*(a2*q3d^2*sin(q3) - a3*cos(q2 + q3)*(q2dd + q3dd) + a3*sin(q2 + q3)*(q2d + q3d)^2 - a2*q3dd*cos(q3)) - q1ddd*(a3*sin(q2 + q3) + a2*sin(q3)) - q2ddd*(a3*sin(q2 + q3) + a2*sin(q3)) - q3ddd*(a3*sin(q2 + q3) + a2*sin(q3));
                                                                                                                                             2*q1dd*(a3*cos(q2 + q3)*(q2d + q3d) + a5*q2d*cos(q2)) - q1d*(a5*q2d^2*sin(q2) - a3*cos(q2 + q3)*(q2dd + q3dd) + a3*sin(q2 + q3)*(q2d + q3d)^2 - a5*q2dd*cos(q2)) + q1ddd*(a3*sin(q2 + q3) + a5*sin(q2)) + a2*q3d^3*sin(q3) - a2*q3ddd*sin(q3) - 3*a2*q3d*q3dd*cos(q3),                                                                                                                                                                                                                                                                                                                                                                                                                                                                                                                                                                 a2*sin(q3)*q3d^3 - 3*a2*q3dd*cos(q3)*q3d - a2*q3ddd*sin(q3),                                                                                                                                                                                                                                                                                                                                                                                 a2*q3d^3*sin(q3) - a2*q1ddd*sin(q3) - a2*q2ddd*sin(q3) - a2*q3ddd*sin(q3) - a2*q1d*q3dd*cos(q3) - 2*a2*q3d*q1dd*cos(q3) - a2*q2d*q3dd*cos(q3) - 2*a2*q3d*q2dd*cos(q3) - 3*a2*q3d*q3dd*cos(q3) + a2*q1d*q3d^2*sin(q3) + a2*q2d*q3d^2*sin(q3);
                                                                                                                   2*q1dd*(a3*cos(q2 + q3)*(q2d + q3d) + a2*q3d*cos(q3)) - q1d*(a2*q3d^2*sin(q3) - a3*cos(q2 + q3)*(q2dd + q3dd) + a3*sin(q2 + q3)*(q2d + q3d)^2 - a2*q3dd*cos(q3)) + q1ddd*(a3*sin(q2 + q3) + a2*sin(q3)) + a2*q2ddd*sin(q3) + a2*q2d*q3dd*cos(q3) + 2*a2*q3d*q2dd*cos(q3) - a2*q2d*q3d^2*sin(q3),                                                                                                                                                                                                                                                                                                                                                                                                                                               a2*q1ddd*sin(q3) + a2*q2ddd*sin(q3) + a2*q1d*q3dd*cos(q3) + 2*a2*q3d*q1dd*cos(q3) + a2*q2d*q3dd*cos(q3) + 2*a2*q3d*q2dd*cos(q3) - a2*q1d*q3d^2*sin(q3) - a2*q2d*q3d^2*sin(q3),                                                                                                                                                                                                                                                                                                                                                                                                                                                                                                                                                                                                                           0];

%% Derivatives of the gravity term

l1 = 1;
l2 = 1;

dotg = [ - g0*m2*(l1*q1d*sin(q1) + d2*sin(q1 + q2)*(q1d + q2d)) - g0*m3*(l1*q1d*sin(q1) + d3*sin(q1 + q2 + q3)*(q1d + q2d + q3d) + l2*sin(q1 + q2)*(q1d + q2d)) - d1*g0*m1*q1d*sin(q1);
                                                            - g0*m3*(d3*sin(q1 + q2 + q3)*(q1d + q2d + q3d) + l2*sin(q1 + q2)*(q1d + q2d)) - d2*g0*m2*sin(q1 + q2)*(q1d + q2d);
                                                                                                                                 -d3*g0*m3*sin(q1 + q2 + q3)*(q1d + q2d + q3d)];

ddotg = [- g0*m2*(l1*q1dd*sin(q1) + l1*q1d^2*cos(q1) + d2*sin(q1 + q2)*(q1dd + q2dd) + d2*cos(q1 + q2)*(q1d + q2d)^2) - g0*m3*(l1*q1dd*sin(q1) + d3*sin(q1 + q2 + q3)*(q1dd + q2dd + q3dd) + l1*q1d^2*cos(q1) + l2*sin(q1 + q2)*(q1dd + q2dd) + d3*cos(q1 + q2 + q3)*(q1d + q2d + q3d)^2 + l2*cos(q1 + q2)*(q1d + q2d)^2) - d1*g0*m1*q1d^2*cos(q1) - d1*g0*m1*q1dd*sin(q1);
                                                                                                                        - g0*m3*(d3*sin(q1 + q2 + q3)*(q1dd + q2dd + q3dd) + l2*sin(q1 + q2)*(q1dd + q2dd) + d3*cos(q1 + q2 + q3)*(q1d + q2d + q3d)^2 + l2*cos(q1 + q2)*(q1d + q2d)^2) - d2*g0*m2*sin(q1 + q2)*(q1dd + q2dd) - d2*g0*m2*cos(q1 + q2)*(q1d + q2d)^2;
                                                                                                                                                                                 - d3*g0*m3*sin(q1 + q2 + q3)*(q1dd + q2dd + q3dd) - d3*g0*m3*cos(q1 + q2 + q3)*(q1d + q2d + q3d)^2];

%% Derivation of u_ESP_invhat

% first we compute the time derivative of:
% a = -invK1*D*ddot_q_tilda-invK1*K2*q_dot+invK1*dot_g+K1*dot_q

%N_dot = dotg - D*ddot_q_tilda + dotM*qd_2dot + M*qd_3dot + dotC*qd_dot + C*qd_2dot;
%N_2dot = ddotg - D*dddot_q_tilda + ddotM*qd_2dot + 2*dotM*qd_3dot + M*qd_4dot + ddotC*qd_dot + 2*dotC*qd_2dot + C*qd_3dot;

%Gamma = -K2*dot_q_tilda + N_dot;
%Gamma_dot = -(dotK2*dot_q_tilda + K2*ddot_q_tilda) + N_2dot;

%a_dot = ddot_q_tilda + qd_2dot + dotinvK1*Gamma + invK1*Gamma_dot;

a_dot = -invK1*D*dddot_q_tilda - invK1*K2*qd_2dot + invK1*ddotg + K1*qd_2dot;

% control
u_ESPp_invhat = B*a_dot;
